simulink model "CIGRE_Networks"  (R2022b)
settings: Solver=VariableStepAuto  StartTime=0.0  StopTime=2  RelTol=1e-3
libraries: spsThreePhasePISectionLineLib x15, spsThreePhaseVIMeasurementLib x14, spsThreePhaseBreakerLib x3, spsThreePhaseSourceLib x2, spsThreePhaseTransformerTwoWindingsLib x2, ee_lib x1, sps_lib x1
settings Model: Creator=r.dong  LastModifiedBy=r.dong

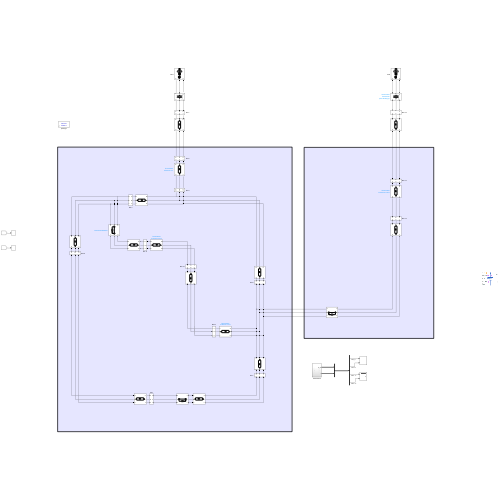
[thumbnail: Simulink's stored preview of the top-level diagram]
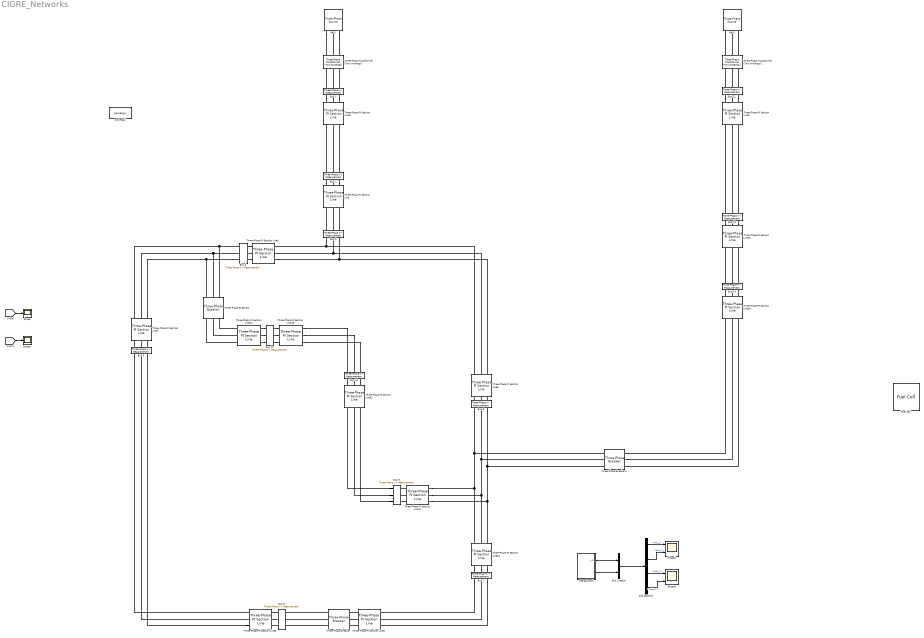
== system CIGRE_Networks ==
  Bus Creator : BusCreator  Inputs=2
  Bus Selector : BusSelector  OutputSignals=I.Iabc_1,I.Iabc_2,U.Vabc_1,U.Vabc_2
  Bus 1 : spsThreePhaseVIMeasurementLib/Three-Phase V-I Measurement  VoltageMeasurement=phase-to-phase  SetLabelV=on  LabelV=Vabc_1  Vpu=off  VpuLL=off  CurrentMeasurement=yes  SetLabelI=on  LabelI=Iabc_1  Ipu=off  Pbase=100e6  Vbase=500e3  OutputType=Complex  PhasorSimulation=off  PSBequivalent=0
  Bus 10 : spsThreePhaseVIMeasurementLib/Three-Phase V-I Measurement  VoltageMeasurement=phase-to-phase  SetLabelV=on  LabelV=Vabc_10  Vpu=off  VpuLL=off  CurrentMeasurement=yes  SetLabelI=on  LabelI=Iabc_10  Ipu=off  Pbase=100e6  Vbase=500e3  OutputType=Complex  PhasorSimulation=off  PSBequivalent=0
  Bus 11 : spsThreePhaseVIMeasurementLib/Three-Phase V-I Measurement  VoltageMeasurement=phase-to-phase  SetLabelV=on  LabelV=Vabc_11  Vpu=off  VpuLL=off  CurrentMeasurement=yes  SetLabelI=on  LabelI=Iabc_11  Ipu=off  Pbase=100e6  Vbase=500e3  OutputType=Complex  PhasorSimulation=off  PSBequivalent=0
  Bus 12 : spsThreePhaseVIMeasurementLib/Three-Phase V-I Measurement  VoltageMeasurement=phase-to-phase  SetLabelV=on  LabelV=Vabc_12  Vpu=off  VpuLL=off  CurrentMeasurement=yes  SetLabelI=on  LabelI=Iabc_12  Ipu=off  Pbase=100e6  Vbase=500e3  OutputType=Complex  PhasorSimulation=off  PSBequivalent=0
  Bus 13 : spsThreePhaseVIMeasurementLib/Three-Phase V-I Measurement  VoltageMeasurement=phase-to-phase  SetLabelV=on  LabelV=Vabc_13  Vpu=off  VpuLL=off  CurrentMeasurement=yes  SetLabelI=on  LabelI=Iabc_13  Ipu=off  Pbase=100e6  Vbase=500e3  OutputType=Complex  PhasorSimulation=off  PSBequivalent=0
  Bus 14 : spsThreePhaseVIMeasurementLib/Three-Phase V-I Measurement  VoltageMeasurement=phase-to-phase  SetLabelV=on  LabelV=Vabc_14  Vpu=off  VpuLL=off  CurrentMeasurement=yes  SetLabelI=on  LabelI=Iabc_14  Ipu=off  Pbase=100e6  Vbase=500e3  OutputType=Complex  PhasorSimulation=off  PSBequivalent=0
  Bus 2 : spsThreePhaseVIMeasurementLib/Three-Phase V-I Measurement  VoltageMeasurement=phase-to-phase  SetLabelV=on  LabelV=Vabc_2  Vpu=off  VpuLL=off  CurrentMeasurement=yes  SetLabelI=on  LabelI=Iabc_2  Ipu=off  Pbase=100e6  Vbase=500e3  OutputType=Complex  PhasorSimulation=off  PSBequivalent=0
  Bus 3 : spsThreePhaseVIMeasurementLib/Three-Phase V-I Measurement  VoltageMeasurement=phase-to-ground  SetLabelV=on  LabelV=Vabc_3  Vpu=off  VpuLL=off  CurrentMeasurement=yes  SetLabelI=on  LabelI=Iabc_3  Ipu=off  Pbase=100e6  Vbase=500e3  OutputType=Complex  PhasorSimulation=off  PSBequivalent=0
  Bus 4 : spsThreePhaseVIMeasurementLib/Three-Phase V-I Measurement  VoltageMeasurement=phase-to-phase  SetLabelV=on  LabelV=Vabc_4  Vpu=off  VpuLL=off  CurrentMeasurement=yes  SetLabelI=on  LabelI=Iabc_4  Ipu=off  Pbase=100e6  Vbase=500e3  OutputType=Complex  PhasorSimulation=off  PSBequivalent=0
  Bus 5 : spsThreePhaseVIMeasurementLib/Three-Phase V-I Measurement  VoltageMeasurement=phase-to-phase  SetLabelV=on  LabelV=Vabc_5  Vpu=off  VpuLL=off  CurrentMeasurement=yes  SetLabelI=on  LabelI=Iabc_5  Ipu=off  Pbase=100e6  Vbase=500e3  OutputType=Complex  PhasorSimulation=off  PSBequivalent=0
  Bus 6 : spsThreePhaseVIMeasurementLib/Three-Phase V-I Measurement  VoltageMeasurement=phase-to-phase  SetLabelV=on  LabelV=Vabc_6  Vpu=off  VpuLL=off  CurrentMeasurement=yes  SetLabelI=on  LabelI=Iabc_6  Ipu=off  Pbase=100e6  Vbase=500e3  OutputType=Complex  PhasorSimulation=off  PSBequivalent=0
  Bus 7 : spsThreePhaseVIMeasurementLib/Three-Phase V-I Measurement  VoltageMeasurement=phase-to-phase  SetLabelV=on  LabelV=Vabc_7  Vpu=off  VpuLL=off  CurrentMeasurement=yes  SetLabelI=on  LabelI=Iabc_7  Ipu=off  Pbase=100e6  Vbase=500e3  OutputType=Complex  PhasorSimulation=off  PSBequivalent=0
  Bus 8 : spsThreePhaseVIMeasurementLib/Three-Phase V-I Measurement  VoltageMeasurement=phase-to-phase  SetLabelV=on  LabelV=Vabc_8  Vpu=off  VpuLL=off  CurrentMeasurement=yes  SetLabelI=on  LabelI=Iabc_8  Ipu=off  Pbase=100e6  Vbase=500e3  OutputType=Complex  PhasorSimulation=off  PSBequivalent=0
  Bus 9 : spsThreePhaseVIMeasurementLib/Three-Phase V-I Measurement  VoltageMeasurement=phase-to-phase  SetLabelV=on  LabelV=Vabc_9  Vpu=off  VpuLL=off  CurrentMeasurement=yes  SetLabelI=on  LabelI=Iabc_9  Ipu=off  Pbase=100e6  Vbase=500e3  OutputType=Complex  PhasorSimulation=off  PSBequivalent=0
  Fuel Cell : ee_lib/Sources/Fuel Cell  model_fidelity=ee.enum.fuelcell.fidelity.detailed  Eoc=65 V  A=0.23 V  ri=0.05 Ohm  i0=80 A  i_lim=200 A  N_cell=65  number_unit=10  pH2_nom=1.5e5 Pa  pO2_nom=1.0e5 Pa  xH2=99  xO2=21  xW=1  dyn=ee.enum.include.no  Rd=0.005 Ohm  tau=10 s  Tnom=293.15 K  thermal_mass=30000 J/K  iFC_specify=off  iFC_priority=None  iFC=0 A  iFC_nominal_specify=off  iFC_nominal_unit=A  iFC_nominal_value=1  vFC_specify=off  vFC_priority=None  vFC=0 V  vFC_nominal_specify=off  vFC_nominal_unit=V  vFC_nominal_value=1  temperature_specify=off  temperature_priority=High  temperature=293 K  temperature_nominal_specify=off  temperature_nominal_unit=K  temperature_nominal_value=1
      settings: InternalSimscapePortConfiguration="{\"Bottom\":[],\"Left\":[{\"id\":\"H\",\"label\":\"H\",\"type\":\"foundation.thermal.thermal\"},{\"id\":\"pfuel\",\"label\":\"pfuel\",\"type\":\"input\"},{\"id\":\"pair\",\"label\":\"pair\",\"type\":\"input\"},{\"id\":\"qfuel\",\"label\":\"qfuel\",\"type\":\"input\"},{\"id\":\"qair\",\"label\":\"qair\",\"type\":\"input\"}],\"Right\":[{\"id\":\"p\",\"label\":\"+\",\"type\":\"foundation.electrical.electrical\"},{\"id\":\"n\",\"label\":\"-\",\"type\":\"foundation.electrical.electrical\"}],\"Top\":[]}"
  Gen1 : spsThreePhaseSourceLib/Three-Phase Source  InternalConnection=Yg  VoltagePhases=off  Voltage=1.06  PhaseAngle=0  Voltage_phases=[25e3 25e3 25e3]/sqrt(3)  PhaseAngles_phases=[0 -120 +120]  Frequency=50  NonIdealSource=on  SpecifyImpedance=on  Resistance=0.8929  Inductance=16.58e-3  ShortCircuitLevel=100e6  BaseVoltage=1  XRratio=1  BusType=swing  Pref=10e3  Qref=0  Prefabc=[10e3, 10e3, 10e3]  Qrefabc=[0, 0, 0]  Qmin=-inf  Qmax=inf
  Gen2 : spsThreePhaseSourceLib/Three-Phase Source  InternalConnection=Yg  VoltagePhases=off  Voltage=1.06  PhaseAngle=0  Voltage_phases=[25e3 25e3 25e3]/sqrt(3)  PhaseAngles_phases=[0 -120 +120]  Frequency=50  NonIdealSource=on  SpecifyImpedance=on  Resistance=0.8929  Inductance=16.58e-3  ShortCircuitLevel=100e6  BaseVoltage=1  XRratio=1  BusType=swing  Pref=10e3  Qref=0  Prefabc=[10e3, 10e3, 10e3]  Qrefabc=[0, 0, 0]  Qmin=-inf  Qmax=inf
  Scope : Scope
  Scope1 : Scope
  Scope2 : Scope  NumInputPorts=2
  Scope3 : Scope  NumInputPorts=2
  Three-Phase PI Section Line{,6,11,14} (4 alike) : spsThreePhasePISectionLineLib/Three-Phase PI Section Line  LConnTagsString=a|b|c  RConnTagsString=A|B|C  Length=4.4  Frequency=50  Resistances=[ 0.01273 0.3864]  Inductances="[ 0.9337e-3  4.1264e-3]"  Capacitances=[12.74e-9 7.751e-9]
  Three-Phase PI Section Line10 : spsThreePhasePISectionLineLib/Three-Phase PI Section Line  LConnTagsString=a|b|c  RConnTagsString=A|B|C  Length=1.7  Frequency=50  Resistances=[ 0.01273 0.3864]  Inductances="[ 0.9337e-3  4.1264e-3]"  Capacitances=[12.74e-9 7.751e-9]
  Three-Phase PI Section Line12 : spsThreePhasePISectionLineLib/Three-Phase PI Section Line  LConnTagsString=a|b|c  RConnTagsString=A|B|C  Length=0.8  Frequency=50  Resistances=[ 0.01273 0.3864]  Inductances="[ 0.9337e-3  4.1264e-3]"  Capacitances=[12.74e-9 7.751e-9]
  Three-Phase PI Section Line13 : spsThreePhasePISectionLineLib/Three-Phase PI Section Line  LConnTagsString=a|b|c  RConnTagsString=A|B|C  Length=0.3  Frequency=50  Resistances=[ 0.01273 0.3864]  Inductances="[ 0.9337e-3  4.1264e-3]"  Capacitances=[12.74e-9 7.751e-9]
  Three-Phase PI Section Line15 : spsThreePhasePISectionLineLib/Three-Phase PI Section Line  LConnTagsString=a|b|c  RConnTagsString=A|B|C  Length=3  Frequency=50  Resistances=[ 0.01273 0.3864]  Inductances="[ 0.9337e-3  4.1264e-3]"  Capacitances=[12.74e-9 7.751e-9]
  Three-Phase PI Section Line16 : spsThreePhasePISectionLineLib/Three-Phase PI Section Line  LConnTagsString=a|b|c  RConnTagsString=A|B|C  Length=2  Frequency=50  Resistances=[ 0.01273 0.3864]  Inductances="[ 0.9337e-3  4.1264e-3]"  Capacitances=[12.74e-9 7.751e-9]
  Three-Phase PI Section Line2 : spsThreePhasePISectionLineLib/Three-Phase PI Section Line  LConnTagsString=a|b|c  RConnTagsString=A|B|C  Length=4.9  Frequency=50  Resistances=[ 0.01273 0.3864]  Inductances="[ 0.9337e-3  4.1264e-3]"  Capacitances=[12.74e-9 7.751e-9]
  Three-Phase PI Section Line3 : spsThreePhasePISectionLineLib/Three-Phase PI Section Line  LConnTagsString=a|b|c  RConnTagsString=A|B|C  Length=2.8  Frequency=50  Resistances=[ 0.01273 0.3864]  Inductances="[ 0.9337e-3  4.1264e-3]"  Capacitances=[12.74e-9 7.751e-9]
  Three-Phase PI Section Line5 : spsThreePhasePISectionLineLib/Three-Phase PI Section Line  LConnTagsString=a|b|c  RConnTagsString=A|B|C  Length=0.6  Frequency=50  Resistances=[ 0.01273 0.3864]  Inductances="[ 0.9337e-3  4.1264e-3]"  Capacitances=[12.74e-9 7.751e-9]
  Three-Phase PI Section Line7 : spsThreePhasePISectionLineLib/Three-Phase PI Section Line  LConnTagsString=a|b|c  RConnTagsString=A|B|C  Length=0.6  Frequency=50  Resistances=[ 0.01273 0.3864]  Inductances="[ 0.9337e-3  4.1264e-3]"  Capacitances=[12.74e-9 7.751e-9]
  Three-Phase PI Section Line8 : spsThreePhasePISectionLineLib/Three-Phase PI Section Line  LConnTagsString=a|b|c  RConnTagsString=A|B|C  Length=1.5  Frequency=50  Resistances=[ 0.01273 0.3864]  Inductances="[ 0.9337e-3  4.1264e-3]"  Capacitances=[12.74e-9 7.751e-9]
  Three-Phase PI Section Line9 : spsThreePhasePISectionLineLib/Three-Phase PI Section Line  LConnTagsString=a|b|c  RConnTagsString=A|B|C  Length=0.2  Frequency=50  Resistances=[ 0.01273 0.3864]  Inductances="[ 0.9337e-3  4.1264e-3]"  Capacitances=[12.74e-9 7.751e-9]
  Three-Phase Transformer (Two Windings) : spsThreePhaseTransformerTwoWindingsLib/Three-Phase Transformer (Two Windings)  Winding1Connection=Yg  Winding2Connection=Yg  CoreType=Three single-phase transformers  SetSaturation=off  Hysteresis=off  DataFile='hysteresis'  SetInitialFlux=off  Measurements=None  UNITS=pu  NominalPower=[ 1 , 50 ]  Winding1=[1.06 , 0.002 , 0.08 ]  Winding2=[ 1.06 , 0.002 , 0.08 ]  Rm=500  Lm=500  L0=0.5  Saturation=[ 0,0 ; 0.0024,1.2 ; 1.0,1.52 ]  InitialFluxes=[ 0.8 , -0.8 , 0.7 ]  BreakLoop=off  DiscreteSolver=Trapezoidal iterative  DataType=off  TransfoNumber=1
  Three-Phase Transformer (Two Windings)1 : spsThreePhaseTransformerTwoWindingsLib/Three-Phase Transformer (Two Windings)  Winding1Connection=Yg  Winding2Connection=Yg  CoreType=Three single-phase transformers  SetSaturation=off  Hysteresis=off  DataFile='hysteresis'  SetInitialFlux=off  Measurements=None  UNITS=pu  NominalPower=[ 1 , 50 ]  Winding1=[1.06 , 0.002 , 0.08 ]  Winding2=[ 1.06 , 0.002 , 0.08 ]  Rm=500  Lm=500  L0=0.5  Saturation=[ 0,0 ; 0.0024,1.2 ; 1.0,1.52 ]  InitialFluxes=[ 0.8 , -0.8 , 0.7 ]  BreakLoop=off  DiscreteSolver=Trapezoidal iterative  DataType=off  TransfoNumber=1
  Three-Phase Breaker : spsThreePhaseBreakerLib/Three-Phase Breaker  InitialState=closed  SwitchA=on  SwitchB=on  SwitchC=on  SwitchTimes="[1/60  5/60]"  External=off  BreakerResistance=0.01  SnubberResistance=1e6  SnubberCapacitance=inf  Measurements=None
  Three-Phase Breaker1 : spsThreePhaseBreakerLib/Three-Phase Breaker  InitialState=closed  SwitchA=on  SwitchB=on  SwitchC=on  SwitchTimes="[1/60  5/60]"  External=off  BreakerResistance=0.01  SnubberResistance=1e6  SnubberCapacitance=inf  Measurements=None
  Three-Phase Breaker2 : spsThreePhaseBreakerLib/Three-Phase Breaker  InitialState=closed  SwitchA=on  SwitchB=on  SwitchC=on  SwitchTimes="[1/60  5/60]"  External=off  BreakerResistance=0.01  SnubberResistance=1e6  SnubberCapacitance=inf  Measurements=None
  meseaument : Subsystem
  powergui : sps_lib/powergui  Priority=1  SimulationMode=Discrete  SampleTime=50e-5  frequency=60  Iterations=50  frequencyindice=50  Pbase=100e6  ErrMax=1e-4  UnitsV=kV  UnitsW=MW  buscounter=0  FunctionMessages=off  echomessages=off  EnableUseOfTLC=off  CurrentSourceSwitches=off  DisableSnubberDevices=off  DisableRonSwitches=off  DisableVfSwitches=off  DisplayEquations=off  AutomaticDiscreteSolvers=off  SolverType=Tustin/Backward Euler (TBE)  Interpol=off  ExternalGateDelay=off  methode=off  Ts=100  x0status=blocks  SPID=on  SwTol=0  HookPort=off  NonlinearTolerance=1e-4  nMaxIteration=100  ContinueOnMaxIteration=off  RestoreLinks=warning  ResistiveCurrentMeasurement=off  Frange=[0:2:500]  Ylog=off  Xlog=on  ShowGrid=off  save=off  variable=ZData  structure=0  ZoomFFT=off  StartTime=0.0  cycles=1  DisplayStyle=1  fundamental=60  FreqAxis=off  MaxFrequency=1000  frequencyindicesteady=1  RmsSteady=1  display=off
  wires:
  [Vabc_1] -> Scope/1
  [Vabc_8] -> Scope1/1
  meseaument/2(I) -> Bus Creator/2
  meseaument/1(U_SI) -> Bus Creator/1
  Bus Creator/1 -> Bus Selector/1
  Bus Selector/1 -> Scope2/1  "<Iabc_1>"
  Bus Selector/2 -> Scope2/2  "<Iabc_2>"
  Bus Selector/3 -> Scope3/1  "<Vabc_1>"
  Bus Selector/4 -> Scope3/2  "<Vabc_2>"
  connections:
  Gen1/RConn2 -- Three-Phase Transformer (Two Windings)/LConn2
  Gen1/RConn3 -- Three-Phase Transformer (Two Windings)/LConn3
  Gen1/RConn1 -- Three-Phase Transformer (Two Windings)/LConn1
  Bus 12/RConn3 -- Three-Phase PI Section Line2/LConn3
  Bus 12/RConn1 -- Three-Phase PI Section Line2/LConn1
  Bus 12/LConn3 -- Three-Phase Transformer (Two Windings)1/RConn3
  Bus 12/LConn2 -- Three-Phase Transformer (Two Windings)1/RConn2
  Bus 12/RConn2 -- Three-Phase PI Section Line2/LConn2
  Gen2/RConn1 -- Three-Phase Transformer (Two Windings)1/LConn1
  Gen2/RConn3 -- Three-Phase Transformer (Two Windings)1/LConn3
  Bus 12/LConn1 -- Three-Phase Transformer (Two Windings)1/RConn1
  Gen2/RConn2 -- Three-Phase Transformer (Two Windings)1/LConn2
  Bus 1/LConn1 -- Three-Phase Transformer (Two Windings)/RConn1
  Bus 1/LConn2 -- Three-Phase Transformer (Two Windings)/RConn2
  Bus 1/LConn3 -- Three-Phase Transformer (Two Windings)/RConn3
  Bus 1/RConn1 -- Three-Phase PI Section Line3/LConn1
  Bus 1/RConn2 -- Three-Phase PI Section Line3/LConn2
  Bus 1/RConn3 -- Three-Phase PI Section Line3/LConn3
  Bus 2/LConn1 -- Three-Phase PI Section Line3/RConn1
  Bus 2/LConn2 -- Three-Phase PI Section Line3/RConn2
  Bus 2/LConn3 -- Three-Phase PI Section Line3/RConn3
  Bus 2/RConn1 -- Three-Phase PI Section Line/LConn1
  Bus 2/RConn2 -- Three-Phase PI Section Line/LConn2
  Bus 2/RConn3 -- Three-Phase PI Section Line/LConn3
  Bus 3/LConn1 -- Three-Phase PI Section Line/RConn1
  Bus 3/LConn2 -- Three-Phase PI Section Line/RConn2
  Bus 3/LConn3 -- Three-Phase PI Section Line/RConn3
  Bus 3/RConn1 -- Three-Phase PI Section Line6/LConn1 -- Three-Phase PI Section Line5/LConn1
  Three-Phase PI Section Line5/LConn2 -- Three-Phase PI Section Line6/LConn2 -- Bus 3/RConn2
  Three-Phase PI Section Line5/LConn3 -- Three-Phase PI Section Line6/LConn3 -- Bus 3/RConn3
  Bus 4/LConn1 -- Three-Phase PI Section Line5/RConn1
  Bus 4/LConn2 -- Three-Phase PI Section Line5/RConn2
  Bus 4/LConn3 -- Three-Phase PI Section Line5/RConn3
  Bus 5/LConn3 -- Three-Phase PI Section Line7/RConn3
  Bus 5/LConn2 -- Three-Phase PI Section Line7/RConn2
  Bus 5/LConn1 -- Three-Phase PI Section Line7/RConn1
  Three-Phase PI Section Line7/LConn1 -- Bus 4/RConn1 -- Three-Phase Breaker1/LConn1
  Three-Phase PI Section Line7/LConn2 -- Bus 4/RConn2 -- Three-Phase Breaker1/LConn2
  Three-Phase PI Section Line7/LConn3 -- Bus 4/RConn3 -- Three-Phase Breaker1/LConn3
  Bus 6/LConn1 -- Three-Phase PI Section Line8/RConn1
  Bus 6/LConn2 -- Three-Phase PI Section Line8/RConn2
  Bus 6/LConn3 -- Three-Phase PI Section Line8/RConn3
  Bus 5/RConn1 -- Three-Phase PI Section Line8/LConn1
  Bus 5/RConn2 -- Three-Phase PI Section Line8/LConn2
  Three-Phase PI Section Line8/LConn3 -- Bus 5/RConn3
  Three-Phase Breaker/LConn1 -- Bus 6/RConn1
  Three-Phase Breaker/LConn2 -- Bus 6/RConn2
  Three-Phase Breaker/LConn3 -- Bus 6/RConn3
  Bus 7/LConn3 -- Three-Phase PI Section Line9/RConn3
  Bus 7/LConn2 -- Three-Phase PI Section Line9/RConn2
  Bus 7/LConn1 -- Three-Phase PI Section Line9/RConn1
  Three-Phase PI Section Line9/LConn1 -- Three-Phase Breaker/RConn1
  Three-Phase PI Section Line9/LConn2 -- Three-Phase Breaker/RConn2
  Three-Phase PI Section Line9/LConn3 -- Three-Phase Breaker/RConn3
  Bus 8/LConn2 -- Three-Phase Breaker2/RConn2 -- Three-Phase PI Section Line10/RConn2 -- Three-Phase PI Section Line11/LConn2
  Bus 8/LConn1 -- Three-Phase Breaker2/RConn1 -- Three-Phase PI Section Line10/RConn1 -- Three-Phase PI Section Line11/LConn1
  Bus 8/LConn3 -- Three-Phase Breaker2/RConn3 -- Three-Phase PI Section Line10/RConn3 -- Three-Phase PI Section Line11/LConn3
  Three-Phase PI Section Line10/LConn1 -- Bus 7/RConn1
  Three-Phase PI Section Line10/LConn2 -- Bus 7/RConn2
  Three-Phase PI Section Line10/LConn3 -- Bus 7/RConn3
  Three-Phase PI Section Line6/RConn1 -- Bus 8/RConn1
  Three-Phase PI Section Line6/RConn2 -- Bus 8/RConn2
  Three-Phase PI Section Line6/RConn3 -- Bus 8/RConn3
  Three-Phase PI Section Line11/RConn2 -- Bus 9/RConn2
  Three-Phase PI Section Line11/RConn1 -- Bus 9/RConn1
  Three-Phase PI Section Line11/RConn3 -- Bus 9/RConn3
  Bus 10/LConn1 -- Three-Phase PI Section Line12/RConn1
  Bus 10/LConn2 -- Three-Phase PI Section Line12/RConn2
  Bus 10/LConn3 -- Three-Phase PI Section Line12/RConn3
  Bus 9/LConn1 -- Three-Phase PI Section Line12/LConn1
  Bus 9/LConn2 -- Three-Phase PI Section Line12/LConn2
  Bus 9/LConn3 -- Three-Phase PI Section Line12/LConn3
  Bus 11/LConn3 -- Three-Phase PI Section Line13/RConn3
  Bus 11/LConn2 -- Three-Phase PI Section Line13/RConn2
  Bus 11/LConn1 -- Three-Phase PI Section Line13/RConn1
  Three-Phase PI Section Line13/LConn1 -- Bus 10/RConn1
  Three-Phase PI Section Line13/LConn2 -- Bus 10/RConn2
  Three-Phase PI Section Line13/LConn3 -- Bus 10/RConn3
  Three-Phase PI Section Line14/LConn1 -- Bus 11/RConn1
  Three-Phase PI Section Line14/LConn2 -- Bus 11/RConn2
  Three-Phase PI Section Line14/LConn3 -- Bus 11/RConn3
  Three-Phase PI Section Line14/RConn1 -- Three-Phase Breaker1/RConn1
  Three-Phase PI Section Line14/RConn2 -- Three-Phase Breaker1/RConn2
  Three-Phase PI Section Line14/RConn3 -- Three-Phase Breaker1/RConn3
  Bus 13/LConn1 -- Three-Phase PI Section Line2/RConn1
  Bus 13/LConn2 -- Three-Phase PI Section Line2/RConn2
  Bus 13/LConn3 -- Three-Phase PI Section Line2/RConn3
  Bus 13/RConn1 -- Three-Phase PI Section Line15/LConn1
  Bus 13/RConn2 -- Three-Phase PI Section Line15/LConn2
  Bus 13/RConn3 -- Three-Phase PI Section Line15/LConn3
  Bus 14/LConn1 -- Three-Phase PI Section Line15/RConn1
  Bus 14/LConn2 -- Three-Phase PI Section Line15/RConn2
  Bus 14/LConn3 -- Three-Phase PI Section Line15/RConn3
  Three-Phase PI Section Line16/LConn1 -- Bus 14/RConn1
  Three-Phase PI Section Line16/LConn2 -- Bus 14/RConn2
  Three-Phase PI Section Line16/LConn3 -- Bus 14/RConn3
  Three-Phase Breaker2/LConn2 -- Three-Phase PI Section Line16/RConn2
  Three-Phase Breaker2/LConn1 -- Three-Phase PI Section Line16/RConn1
  Three-Phase Breaker2/LConn3 -- Three-Phase PI Section Line16/RConn3

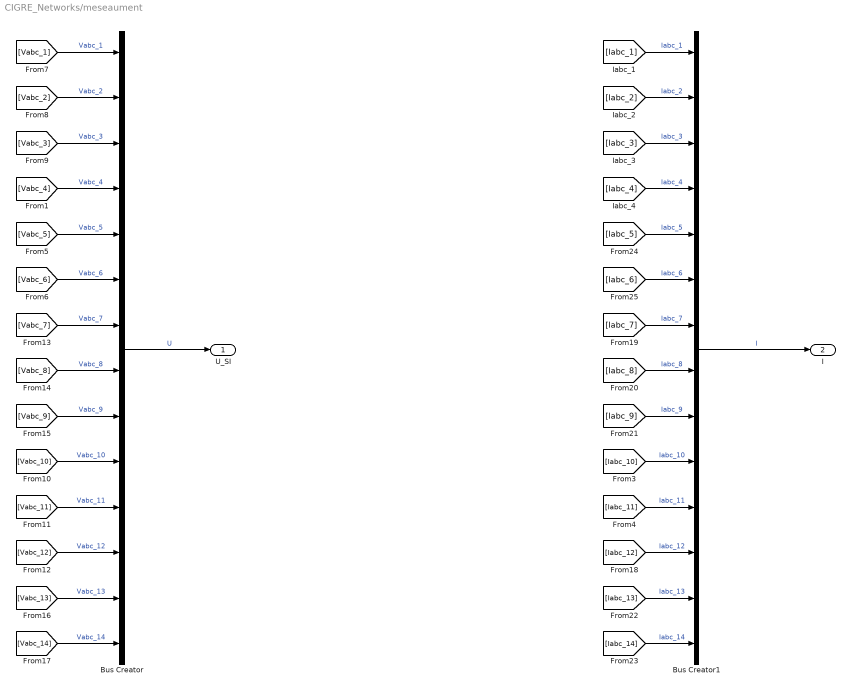
== system CIGRE_Networks/meseaument ==
  Bus Creator : BusCreator  Inputs=14
  Bus Creator1 : BusCreator  Inputs=14
  U_SI : Outport
  I : Outport  Port=2
  wires:
  [Vabc_5] -> Bus Creator/5  "Vabc_5"
  [Vabc_6] -> Bus Creator/6  "Vabc_6"
  [Vabc_7] -> Bus Creator/7  "Vabc_7"
  [Vabc_8] -> Bus Creator/8  "Vabc_8"
  [Vabc_9] -> Bus Creator/9  "Vabc_9"
  [Vabc_10] -> Bus Creator/10  "Vabc_10"
  [Vabc_11] -> Bus Creator/11  "Vabc_11"
  [Vabc_12] -> Bus Creator/12  "Vabc_12"
  [Vabc_13] -> Bus Creator/13  "Vabc_13"
  [Vabc_14] -> Bus Creator/14  "Vabc_14"
  [Vabc_1] -> Bus Creator/1  "Vabc_1"
  [Vabc_2] -> Bus Creator/2  "Vabc_2"
  [Vabc_3] -> Bus Creator/3  "Vabc_3"
  [Vabc_4] -> Bus Creator/4  "Vabc_4"
  [Iabc_1] -> Bus Creator1/1  "Iabc_1"
  [Iabc_2] -> Bus Creator1/2  "Iabc_2"
  [Iabc_3] -> Bus Creator1/3  "Iabc_3"
  [Iabc_4] -> Bus Creator1/4  "Iabc_4"
  [Iabc_5] -> Bus Creator1/5  "Iabc_5"
  [Iabc_6] -> Bus Creator1/6  "Iabc_6"
  [Iabc_7] -> Bus Creator1/7  "Iabc_7"
  [Iabc_8] -> Bus Creator1/8  "Iabc_8"
  [Iabc_9] -> Bus Creator1/9  "Iabc_9"
  [Iabc_10] -> Bus Creator1/10  "Iabc_10"
  [Iabc_11] -> Bus Creator1/11  "Iabc_11"
  [Iabc_12] -> Bus Creator1/12  "Iabc_12"
  [Iabc_13] -> Bus Creator1/13  "Iabc_13"
  [Iabc_14] -> Bus Creator1/14  "Iabc_14"
  Bus Creator/1 -> U_SI/1  "U"
  Bus Creator1/1 -> I/1  "I"
